simulink model "map_test2"  (R2013b)
(part 3 of 114)

  simple_bram_vacc26/1(dout) -> Reinterpret26/1
  simple_bram_vacc27/1(dout) -> Reinterpret27/1
  simple_bram_vacc28/1(dout) -> Reinterpret28/1
  simple_bram_vacc29/1(dout) -> Reinterpret29/1
  Reinterpret26/1 -> pipeline185/1(d)
  Reinterpret27/1 -> pipeline188/1(d)
  Reinterpret28/1 -> pipeline189/1(d)
  Reinterpret29/1 -> pipeline190/1(d)
  Counter10/1 -> Relational18/2, Relational19/2
  Constant64/1 -> Mux29/2
  Constant43/1 -> Mux28/2
  Constant44/1 -> Mux30/2
  Constant45/1 -> Mux31/2
  AddSub17/1 -> AddSub19/1
  AddSub18/1 -> AddSub19/2
  pipeline196/1(q) -> pipeline197/1(d)
  edge_detect5/1 -> Accumulator5/2, Logical11/1
  pipeline195/1(q) -> Accumulator5/3, edge_detect5/1
  Slice6/1 -> Accumulator5/1
  Register5/1 -> frb_detector6/1(out_reg)
  [cnt_rst] -> Register5/2
  Relational17/1 -> Register5/3, Register5/1
  simple_bram_vacc29/2(valid) -> Terminator31/1
  pipeline187/1(q) -> pipeline196/1(d), Mux31/1, Mux30/1, Mux28/1, Logical12/1
  Accumulator5/1 -> Relational17/2, ACC6/2(data_in)
  Counter11/1 -> ACC6/1(addr)
  ACC6/1(data_out) -> Terminator32/1
  Logical11/1 -> Counter11/1
  Delay31/1 -> pipeline191/1(d)
  Delay40/1 -> pipeline192/1(d)
  Delay41/1 -> pipeline193/1(d)
  acc_cntrl5/1(new_acc) -> pipeline186/1(d), pipeline171/1(d), pipeline181/1(d), pipeline174/1(d), pipeline182/1(d)
  pipeline194/1(q) -> pipeline152/1(d)
  pipeline191/1(q) -> pipeline169/1(d)
  pipeline192/1(q) -> pipeline172/1(d)
  pipeline193/1(q) -> pipeline180/1(d)
  pipeline185/1(q) -> Mux29/3
  pipeline188/1(q) -> Mux28/3
  pipeline189/1(q) -> Mux30/3
  pipeline190/1(q) -> Mux31/3
  Mux29/1 -> pipeline199/1(d)
  Mux28/1 -> pipeline200/1(d)
  Mux30/1 -> pipeline201/1(d)
  Mux31/1 -> pipeline202/1(d)
  pipeline199/1(q) -> AddSub17/1
  pipeline200/1(q) -> AddSub17/2
  pipeline201/1(q) -> AddSub18/1
  pipeline202/1(q) -> AddSub18/2
  pipeline197/1(q) -> pipeline195/1(d)
  AddSub19/1 -> Slice6/1
  pipeline141/1(q) -> Logical12/3
  pipeline124/1(q) -> Logical12/2
  Logical12/1 -> Mux29/1
  Relational18/1 -> pipeline124/1(d)
  Relational19/1 -> pipeline141/1(d)
  Constant48/1 -> Relational18/1
  Constant65/1 -> Relational19/1
  Constant38/1 -> Logical11/2, ACC6/3(we)
  theta6/1(in_reg) -> Convert6/1
  Convert6/1 -> Relational17/1
  simple_bram_vacc27/2(valid) -> Terminator30/1
  simple_bram_vacc28/2(valid) -> Terminator29/1
  Delay43/1 -> acc_cntrl6/2(sync)
  [acc_len7] -> acc_cntrl6/1(acc_len)
  [cnt_rst] -> acc_cntrl6/3(rst)
  Delay44/1 -> pipeline234/1(d)
  pipeline215/1(q) -> simple_bram_vacc19/1(new_acc)
  pipeline213/1(q) -> simple_bram_vacc18/1(new_acc)
  pipeline211/1(q) -> simple_bram_vacc31/1(new_acc)
  pipeline218/1(q) -> simple_bram_vacc30/1(new_acc)
  pipeline208/1(q) -> simple_bram_vacc30/2(din)
  pipeline210/1(q) -> simple_bram_vacc31/2(din)
  pipeline212/1(q) -> simple_bram_vacc18/2(din)
  pipeline214/1(q) -> simple_bram_vacc19/2(din)
  pipeline216/1(q) -> Counter12/1
  simple_bram_vacc30/2(valid) -> Counter12/2, pipeline219/1(d)
  simple_bram_vacc30/1(dout) -> Reinterpret30/1
  simple_bram_vacc31/1(dout) -> Reinterpret31/1
  simple_bram_vacc18/1(dout) -> Reinterpret18/1
  simple_bram_vacc19/1(dout) -> Reinterpret19/1
  Reinterpret30/1 -> pipeline217/1(d)
  Reinterpret31/1 -> pipeline220/1(d)
  Reinterpret18/1 -> pipeline222/1(d)
  Reinterpret19/1 -> pipeline225/1(d)
  Counter12/1 -> Relational21/2, Relational22/2
  Constant49/1 -> Mux18/2
  Constant56/1 -> Mux32/2
  Constant57/1 -> Mux19/2
  Constant58/1 -> Mux20/2
  AddSub20/1 -> AddSub22/1
  AddSub21/1 -> AddSub22/2
  pipeline239/1(q) -> pipeline240/1(d)
  edge_detect6/1 -> Accumulator6/2, Logical13/1
  pipeline235/1(q) -> Accumulator6/3, edge_detect6/1
  Slice7/1 -> Accumulator6/1
  Register6/1 -> frb_detector7/1(out_reg)
  [cnt_rst] -> Register6/2
  Relational20/1 -> Register6/3, Register6/1
  simple_bram_vacc19/2(valid) -> Terminator17/1
  pipeline219/1(q) -> pipeline239/1(d), Mux20/1, Mux19/1, Mux32/1, Logical14/1
  Accumulator6/1 -> Relational20/2, ACC7/2(data_in)
  Counter13/1 -> ACC7/1(addr)
  ACC7/1(data_out) -> Terminator19/1
  Logical13/1 -> Counter13/1
  Delay47/1 -> pipeline227/1(d)
  Delay48/1 -> pipeline232/1(d)
  Delay49/1 -> pipeline233/1(d)
  acc_cntrl6/1(new_acc) -> pipeline218/1(d), pipeline211/1(d), pipeline215/1(d), pipeline213/1(d), pipeline216/1(d)
  pipeline234/1(q) -> pipeline208/1(d)
  pipeline227/1(q) -> pipeline210/1(d)
  pipeline232/1(q) -> pipeline212/1(d)
  pipeline233/1(q) -> pipeline214/1(d)
  pipeline217/1(q) -> Mux18/3
  pipeline220/1(q) -> Mux32/3
  pipeline222/1(q) -> Mux19/3
  pipeline225/1(q) -> Mux20/3
  Mux18/1 -> pipeline153/1(d)
  Mux32/1 -> pipeline154/1(d)
  Mux19/1 -> pipeline155/1(d)
  Mux20/1 -> pipeline156/1(d)
  pipeline153/1(q) -> AddSub20/1
  pipeline154/1(q) -> AddSub20/2
  pipeline155/1(q) -> AddSub21/1
  pipeline156/1(q) -> AddSub21/2
  pipeline240/1(q) -> pipeline235/1(d)
  AddSub22/1 -> Slice7/1
  pipeline205/1(q) -> Logical14/3
  pipeline204/1(q) -> Logical14/2
  Logical14/1 -> Mux18/1
  Relational21/1 -> pipeline204/1(d)
  Relational22/1 -> pipeline205/1(d)
  Constant47/1 -> Relational21/1
  Constant50/1 -> Relational22/1
  Constant51/1 -> Logical13/2, ACC7/3(we)
  theta7/1(in_reg) -> Convert7/1
  Convert7/1 -> Relational20/1
  simple_bram_vacc31/2(valid) -> Terminator34/1
  simple_bram_vacc18/2(valid) -> Terminator33/1
  Delay50/1 -> acc_cntrl7/2(sync)
  [acc_len8] -> acc_cntrl7/1(acc_len)
  [cnt_rst] -> acc_cntrl7/3(rst)
  Delay51/1 -> pipeline142/1(d)
  pipeline237/1(q) -> simple_bram_vacc23/1(new_acc)
  pipeline226/1(q) -> simple_bram_vacc22/1(new_acc)
  pipeline223/1(q) -> simple_bram_vacc21/1(new_acc)
  pipeline125/1(q) -> simple_bram_vacc20/1(new_acc)
  pipeline207/1(q) -> simple_bram_vacc20/2(din)
  pipeline221/1(q) -> simple_bram_vacc21/2(din)
  pipeline224/1(q) -> simple_bram_vacc22/2(din)
  pipeline236/1(q) -> simple_bram_vacc23/2(din)
  pipeline238/1(q) -> Counter14/1
  simple_bram_vacc20/2(valid) -> Counter14/2, pipeline126/1(d)
  simple_bram_vacc20/1(dout) -> Reinterpret20/1
  simple_bram_vacc21/1(dout) -> Reinterpret21/1
  simple_bram_vacc22/1(dout) -> Reinterpret22/1
  simple_bram_vacc23/1(dout) -> Reinterpret23/1
  Reinterpret20/1 -> pipeline241/1(d)
  Reinterpret21/1 -> pipeline127/1(d)
  Reinterpret22/1 -> pipeline128/1(d)
  Reinterpret23/1 -> pipeline129/1(d)
  Counter14/1 -> Relational15/2, Relational14/2
  Constant59/1 -> Mux22/2
  Constant52/1 -> Mux21/2
  Constant53/1 -> Mux23/2
  Constant54/1 -> Mux24/2
  AddSub23/1 -> AddSub15/1
  AddSub14/1 -> AddSub15/2
  pipeline144/1(q) -> pipeline145/1(d)
  edge_detect7/1 -> Logical15/1, Accumulator7/2
  pipeline143/1(q) -> Accumulator7/3, edge_detect7/1
  Slice8/1 -> Accumulator7/1
  Register7/1 -> frb_detector8/1(out_reg)
  [cnt_rst] -> Register7/2
  Relational23/1 -> Register7/1, Register7/3
  simple_bram_vacc23/2(valid) -> Terminator24/1
  pipeline126/1(q) -> Logical16/1, Mux21/1, Mux23/1, Mux24/1, pipeline144/1(d)
  Accumulator7/1 -> ACC8/2(data_in), Relational23/2
  Counter15/1 -> ACC8/1(addr)
  ACC8/1(data_out) -> Terminator25/1
  Logical15/1 -> Counter15/1
  Delay42/1 -> pipeline130/1(d)
  Delay45/1 -> pipeline131/1(d)
  Delay46/1 -> pipeline132/1(d)
  acc_cntrl7/1(new_acc) -> pipeline238/1(d), pipeline226/1(d), pipeline237/1(d), pipeline223/1(d), pipeline125/1(d)
  pipeline142/1(q) -> pipeline207/1(d)
  pipeline130/1(q) -> pipeline221/1(d)
  pipeline131/1(q) -> pipeline224/1(d)
  pipeline132/1(q) -> pipeline236/1(d)
  pipeline241/1(q) -> Mux22/3
  pipeline127/1(q) -> Mux21/3
  pipeline128/1(q) -> Mux23/3
  pipeline129/1(q) -> Mux24/3
  Mux22/1 -> pipeline147/1(d)
  Mux21/1 -> pipeline148/1(d)
  Mux23/1 -> pipeline149/1(d)
  Mux24/1 -> pipeline150/1(d)
  pipeline147/1(q) -> AddSub23/1
  pipeline148/1(q) -> AddSub23/2
  pipeline149/1(q) -> AddSub14/1
  pipeline150/1(q) -> AddSub14/2
  pipeline145/1(q) -> pipeline143/1(d)
  AddSub15/1 -> Slice8/1
  pipeline206/1(q) -> Logical16/3
  pipeline203/1(q) -> Logical16/2
  Logical16/1 -> Mux22/1
  Relational14/1 -> pipeline203/1(d)
  Relational15/1 -> pipeline206/1(d)
  Constant55/1 -> Relational14/1
  Constant60/1 -> Relational15/1
  Constant46/1 -> ACC8/3(we), Logical15/2
  theta8/1(in_reg) -> Convert8/1
  Convert8/1 -> Relational23/1
  simple_bram_vacc21/2(valid) -> Terminator23/1
  simple_bram_vacc22/2(valid) -> Terminator20/1
  Delay58/1 -> acc_cntrl8/2(sync)
  [acc_len9] -> acc_cntrl8/1(acc_len)
  [cnt_rst] -> acc_cntrl8/3(rst)
  Delay59/1 -> pipeline290/1(d)
  pipeline275/1(q) -> simple_bram_vacc33/1(new_acc)
  pipeline273/1(q) -> simple_bram_vacc32/1(new_acc)
  pipeline271/1(q) -> simple_bram_vacc39/1(new_acc)
  pipeline278/1(q) -> simple_bram_vacc38/1(new_acc)
  pipeline269/1(q) -> simple_bram_vacc38/2(din)
  pipeline270/1(q) -> simple_bram_vacc39/2(din)
  pipeline272/1(q) -> simple_bram_vacc32/2(din)
  pipeline274/1(q) -> simple_bram_vacc33/2(din)
  pipeline276/1(q) -> Counter16/1
  simple_bram_vacc38/2(valid) -> Counter16/2, pipeline279/1(d)
  simple_bram_vacc38/1(dout) -> Reinterpret38/1
  simple_bram_vacc39/1(dout) -> Reinterpret39/1
  simple_bram_vacc32/1(dout) -> Reinterpret32/1
  simple_bram_vacc33/1(dout) -> Reinterpret33/1
  Reinterpret38/1 -> pipeline277/1(d)
  Reinterpret39/1 -> pipeline280/1(d)
  Reinterpret32/1 -> pipeline282/1(d)
  Reinterpret33/1 -> pipeline285/1(d)
  Counter16/1 -> Relational28/2, Relational27/2
  Constant68/1 -> Mux33/2
  Constant75/1 -> Mux40/2
  Constant76/1 -> Mux34/2
  Constant77/1 -> Mux35/2
  AddSub26/1 -> AddSub28/1
  AddSub27/1 -> AddSub28/2
  pipeline295/1(q) -> pipeline296/1(d)
  edge_detect8/1 -> Logical17/1, Accumulator8/2
  pipeline291/1(q) -> Accumulator8/3, edge_detect8/1
  Slice9/1 -> Accumulator8/1
  Register8/1 -> frb_detector9/1(out_reg)
  [cnt_rst] -> Register8/2
  Relational26/1 -> Register8/1, Register8/3
  simple_bram_vacc33/2(valid) -> Terminator35/1
  pipeline279/1(q) -> Logical18/1, Mux40/1, Mux34/1, Mux35/1, pipeline295/1(d)
  Accumulator8/1 -> ACC9/2(data_in), Relational26/2
  Counter17/1 -> ACC9/1(addr)
  ACC9/1(data_out) -> Terminator36/1
  Logical17/1 -> Counter17/1
  Delay62/1 -> pipeline287/1(d)
  Delay63/1 -> pipeline288/1(d)
  Delay64/1 -> pipeline289/1(d)
  acc_cntrl8/1(new_acc) -> pipeline276/1(d), pipeline273/1(d), pipeline275/1(d), pipeline271/1(d), pipeline278/1(d)
  pipeline290/1(q) -> pipeline269/1(d)
  pipeline287/1(q) -> pipeline270/1(d)
  pipeline288/1(q) -> pipeline272/1(d)
  pipeline289/1(q) -> pipeline274/1(d)
  pipeline277/1(q) -> Mux33/3
  pipeline280/1(q) -> Mux40/3
  pipeline282/1(q) -> Mux34/3
  pipeline285/1(q) -> Mux35/3
  Mux33/1 -> pipeline260/1(d)
  Mux40/1 -> pipeline261/1(d)
  Mux34/1 -> pipeline262/1(d)
  Mux35/1 -> pipeline263/1(d)
  pipeline260/1(q) -> AddSub26/1
  pipeline261/1(q) -> AddSub26/2
  pipeline262/1(q) -> AddSub27/1
  pipeline263/1(q) -> AddSub27/2
  pipeline296/1(q) -> pipeline291/1(d)
  AddSub28/1 -> Slice9/1
  pipeline266/1(q) -> Logical18/3
  pipeline265/1(q) -> Logical18/2
  Logical18/1 -> Mux33/1
  Relational27/1 -> pipeline265/1(d)
  Relational28/1 -> pipeline266/1(d)
  Constant67/1 -> Relational27/1
  Constant69/1 -> Relational28/1
  Constant70/1 -> ACC9/3(we), Logical17/2
  theta9/1(in_reg) -> Convert9/1
  Convert9/1 -> Relational26/1
  simple_bram_vacc39/2(valid) -> Terminator42/1
  simple_bram_vacc32/2(valid) -> Terminator41/1
  Delay65/1 -> acc_cntrl9/2(sync)
  [acc_len10] -> acc_cntrl9/1(acc_len)
  [cnt_rst] -> acc_cntrl9/3(rst)
  Delay66/1 -> pipeline250/1(d)
  pipeline293/1(q) -> simple_bram_vacc37/1(new_acc)
  pipeline286/1(q) -> simple_bram_vacc36/1(new_acc)
  pipeline283/1(q) -> simple_bram_vacc35/1(new_acc)
  pipeline242/1(q) -> simple_bram_vacc34/1(new_acc)
  pipeline268/1(q) -> simple_bram_vacc34/2(din)
  pipeline281/1(q) -> simple_bram_vacc35/2(din)
  pipeline284/1(q) -> simple_bram_vacc36/2(din)
  pipeline292/1(q) -> simple_bram_vacc37/2(din)
  pipeline294/1(q) -> Counter18/1
  simple_bram_vacc34/2(valid) -> Counter18/2, pipeline243/1(d)
  simple_bram_vacc34/1(dout) -> Reinterpret34/1
  simple_bram_vacc35/1(dout) -> Reinterpret35/1
  simple_bram_vacc36/1(dout) -> Reinterpret36/1
  simple_bram_vacc37/1(dout) -> Reinterpret37/1
  Reinterpret34/1 -> pipeline297/1(d)
  Reinterpret35/1 -> pipeline244/1(d)
  Reinterpret36/1 -> pipeline245/1(d)
  Reinterpret37/1 -> pipeline246/1(d)
  Counter18/1 -> Relational24/2, Relational25/2
  Constant78/1 -> Mux37/2
  Constant71/1 -> Mux36/2
  Constant72/1 -> Mux38/2
  Constant73/1 -> Mux39/2
  AddSub29/1 -> AddSub25/1
  AddSub24/1 -> AddSub25/2
  pipeline252/1(q) -> pipeline253/1(d)
  edge_detect9/1 -> Accumulator9/2, Logical19/1
  pipeline251/1(q) -> edge_detect9/1, Accumulator9/3
  Slice10/1 -> Accumulator9/1
  Register9/1 -> frb_detector10/1(out_reg)
  [cnt_rst] -> Register9/2
  Relational29/1 -> Register9/3, Register9/1
  simple_bram_vacc37/2(valid) -> Terminator39/1
  pipeline243/1(q) -> pipeline252/1(d), Mux39/1, Mux38/1, Mux36/1, Logical20/1
  Accumulator9/1 -> Relational29/2, ACC10/2(data_in)
  Counter19/1 -> ACC10/1(addr)
  ACC10/1(data_out) -> Terminator40/1
  Logical19/1 -> Counter19/1
  Delay57/1 -> pipeline247/1(d)
  Delay60/1 -> pipeline248/1(d)
  Delay61/1 -> pipeline249/1(d)
  acc_cntrl9/1(new_acc) -> pipeline242/1(d), pipeline283/1(d), pipeline293/1(d), pipeline286/1(d), pipeline294/1(d)
  pipeline250/1(q) -> pipeline268/1(d)
  pipeline247/1(q) -> pipeline281/1(d)
  pipeline248/1(q) -> pipeline284/1(d)
  pipeline249/1(q) -> pipeline292/1(d)
  pipeline297/1(q) -> Mux37/3
  pipeline244/1(q) -> Mux36/3
  pipeline245/1(q) -> Mux38/3
  pipeline246/1(q) -> Mux39/3
  Mux37/1 -> pipeline255/1(d)
  Mux36/1 -> pipeline256/1(d)
  Mux38/1 -> pipeline257/1(d)
  Mux39/1 -> pipeline258/1(d)
  pipeline255/1(q) -> AddSub29/1
  pipeline256/1(q) -> AddSub29/2
  pipeline257/1(q) -> AddSub24/1
  pipeline258/1(q) -> AddSub24/2
  pipeline253/1(q) -> pipeline251/1(d)
  AddSub25/1 -> Slice10/1
  pipeline267/1(q) -> Logical20/3
  pipeline264/1(q) -> Logical20/2
  Logical20/1 -> Mux37/1
  Relational24/1 -> pipeline264/1(d)
  Relational25/1 -> pipeline267/1(d)
  Constant74/1 -> Relational24/1
  Constant79/1 -> Relational25/1
  Constant66/1 -> Logical19/2, ACC10/3(we)
  theta10/1(in_reg) -> Convert10/1
  Convert10/1 -> Relational29/1
  simple_bram_vacc35/2(valid) -> Terminator38/1
  simple_bram_vacc36/2(valid) -> Terminator37/1
  power7/1 -> Delay15/1, Delay28/1, Delay25/1, Delay54/1, Delay41/1, Delay49/1, Delay46/1, Delay64/1, Delay61/1, Delay122/1, Delay37/1
  power5/1 -> Delay10/1, Delay26/1, Delay18/1, Delay52/1, Delay31/1, Delay47/1, Delay62/1, Delay57/1, Delay120/1, Delay42/1, Delay33/1
  pipeline179/1(q) -> Accumulator4/3, edge_detect4/1
  Constant81/1 -> asiaa_adc5g/1(sim_a)
  Mux2/1 -> pipeline86/1(d)
  Mux1/1 -> pipeline87/1(d)
  Mux3/1 -> pipeline88/1(d)
